simulink model "transientStability_R2013B"  (R2013b)
settings: Solver=ode4  SolverMode=SingleTasking  StartTime=0.0  StopTime=10  FixedStep=0.01  MaxStep=0.01  RelTol=1e-3  AbsTol=1e-2
undefined symbols (not defined in the file): j, mpc
(part 1 of 4)
settings Model: ExtModeTrigMode=oneshot  ExtModeArmWhenConnect=off  Creator=aithal  LastModifiedBy=gelli
settings SolverCC: InitialStep=0.001
settings DataIOCC: LimitDataPoints=off  SignalLoggingSaveFormat=ModelDataLogs  SaveOutput=off  SaveTime=off
settings OptimizationCC: BlockReduction=off  BooleanDataType=off
settings DebuggingCC: SaveWithParameterizedLinksMsg=none  SignalResolutionControl=TryResolveAllWithWarning  SolverPrmCheckMsg=none  MultiTaskDSMMsg=warning  MultiTaskCondExecSysMsg=none  FrameProcessingCompatibilityMsg=error  StateNameClashWarn=warning
settings HardwareCC: TargetUnknown=on
settings GRTTargetCC: CodeReplacementLibrary=C89/C90 (ANSI)  CombineOutputUpdateFcns=off  GRTInterface=on

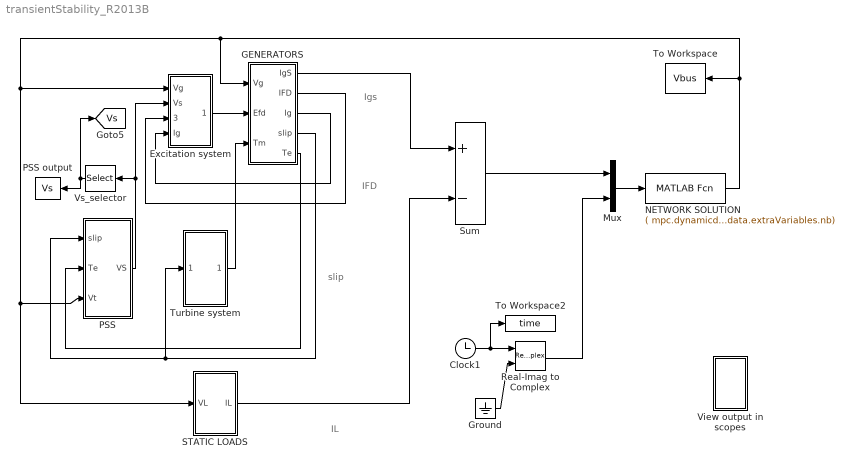
== system transientStability_R2013B ==
  note: Igs
  note: IL
  note: IFD
  note: slip
  Clock1 : Clock
  Excitation system : Subsystem
  GENERATORS : Subsystem
  Ground : Ground
  Mux : Mux  Inputs=[mpc.dynamicdata.extraVariables.nb 1]
  NETWORK SOLUTION : MATLABFcn  MATLABFcn="( mpc.dynamicdata.Yform.Y  * (abs(u(mpc.dynamicdata.extraVariables.nb+1))<mpc.dynamicdata.Yform.Tfault)  + mpc.dynamicdata.Yform.Yf  * (abs(u(mpc.dynamicdata.extraVariables.nb+1))>=mpc.dynamicdata.Yform.Tfault & abs(u(mpc.dynamicdata.extraVariables.nb+1)) <(mpc.dynamicdata.Yform.Tfault+mpc.dynamicdata.Yform.Tclear) ) + mpc.dynamicdata.Yform.Ypf * (abs(u(mpc.dynamicdata.extraVariables.nb+1)) >= (mpc.dynamicdata.Yform.Tfault+mpc.dynamicdata.Yform.Tclear) )  ) \\   u(1:mpc.dynamicdata.extraVariables.nb)"  OutputDimensions=mpc.dynamicdata.extraVariables.nb  OutputSignalType=complex
  PSS : Subsystem
  PSS output : ToWorkspace  VariableName=Vs  SampleTime=0.01
  Real-Imag to Complex : RealImagToComplex
  STATIC LOADS : Subsystem
  Sum : Sum  Inputs=+-  SaturateOnIntegerOverflow=on  InputSameDT=on  OutDataTypeStr=Inherit: Same as first input
  To Workspace : ToWorkspace  VariableName=Vbus  SampleTime=0.01
  To Workspace2 : ToWorkspace  VariableName=time  SampleTime=0.01
  Turbine system : Subsystem
  View output in scopes : Subsystem
  Vs_selector : Selector  InputPortWidth=mpc.dynamicdata.extraVariables.nb  IndexOptions=Index vector (dialog)  Indices=(mpc.dynamicdata.gen(:,1))  OutputSizes=1
  tag scope: Vs=global
  wires:
  Excitation system/1(Efd) -> GENERATORS/2(Efd)
  GENERATORS/2(IFD) -> Excitation system/3(IFD)
  GENERATORS/3(Ig) -> Excitation system/4(Ig)
  GENERATORS/1(IgS) -> Sum/1
  GENERATORS/4(slip) -> Turbine system/1(slip), PSS/1(slip)
  GENERATORS/5(Te) -> PSS/2(Te)
  Sum/1 -> Mux/1
  Ground/1 -> Real-Imag to Complex/2
  Real-Imag to Complex/1 -> Mux/2
  Clock1/1 -> Real-Imag to Complex/1, To Workspace2/1
  Mux/1 -> NETWORK SOLUTION/1
  Turbine system/1(Tm) -> GENERATORS/3(Tm)
  PSS/1(VS) -> Excitation system/2(Vs), Vs_selector/1
  Vs_selector/1 -> PSS output/1, [Vs]
  NETWORK SOLUTION/1 -> GENERATORS/1(Vg), Excitation system/1(Vg), STATIC LOADS/1(VL), PSS/3(Vt), To Workspace/1
  STATIC LOADS/1(IL) -> Sum/2

== system transientStability_R2013B/Excitation system ==
  Vg : Inport
  Vs : Inport  Port=2
  IFD : Inport  Port=3
  Ig : Inport  Port=4
  "Exciter_AC1A " : Subsystem
  Exciter_AC4A : Subsystem
  Exciter_DC1A : Subsystem
  Exciter_ST1A : Subsystem
  Exciter_ST2A : Subsystem
  Exciter_static : Subsystem
  Select-AVR : Subsystem
  Sum1 : Sum  Inputs=++++++  SaturateOnIntegerOverflow=on  InputSameDT=on  OutDataTypeStr=Inherit: Same as first input
  flag : Constant  Value=mpc.dynamicdata.gen_exciterParameters.AVR
  Efd : Outport  InitialOutput=0
  wires:
  Vg/1 -> Exciter_static/1(V), Exciter_DC1A/1(V), Exciter_AC4A/1(V), Exciter_ST2A/1(V), "Exciter_AC1A "/1(V), Exciter_ST1A/1(V)
  Vs/1 -> Exciter_static/2(Vs), Exciter_DC1A/2(Vs), Exciter_AC4A/2(Vs), Exciter_ST2A/2(Vs), "Exciter_AC1A "/2(Vs), Exciter_ST1A/2(Vs)
  Exciter_static/1(Efd) -> Sum1/1
  Exciter_DC1A/1(Efd) -> Sum1/2
  Exciter_AC4A/1(Efd) -> Sum1/3
  Ig/1 -> Exciter_ST2A/4(Ia)
  Exciter_ST2A/1(Efd) -> Sum1/4
  IFD/1 -> Exciter_AC4A/3(IFD), Exciter_ST2A/3(IFD), "Exciter_AC1A "/3(IFD), Exciter_ST1A/3(IFD)
  "Exciter_AC1A "/1(Efd) -> Sum1/5
  Select-AVR/1(out_1) -> Efd/1
  Sum1/1 -> Select-AVR/2(in_2)
  flag/1 -> Select-AVR/1(in_1)
  Exciter_ST1A/1(Efd) -> Sum1/6

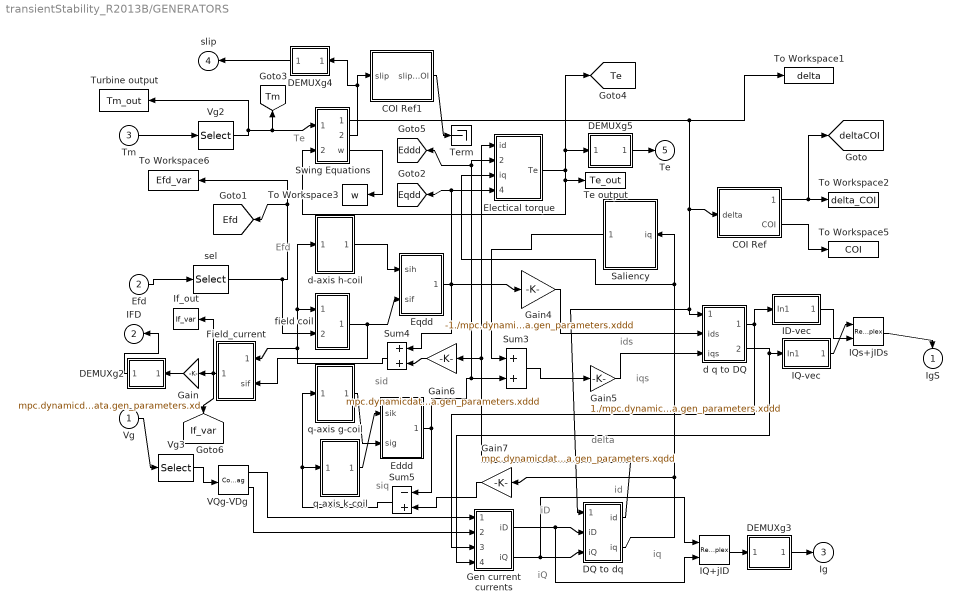
== system transientStability_R2013B/GENERATORS ==
  note: iq
  note: id
  note: Efd
  note: Te
  note: sid
  note: siq
  note: iqs
  note: ids
  note: iD
  note: iQ
  note: delta
  Vg : Inport
  Efd : Inport  Port=2
  Tm : Inport  Port=3
  " field coil" : Subsystem
  COI Ref : Subsystem
  COI Ref1 : Subsystem
  DEMUXg2 : Subsystem
  DEMUXg3 : Subsystem
  DEMUXg4 : Subsystem
  DEMUXg5 : Subsystem
  DQ to dq : Subsystem
  Eddd : Subsystem
  Electical torque : Subsystem
  "Eqdd " : Subsystem
  Field_current : Subsystem
  Gain : Gain  Gain=mpc.dynamicdata.gen_parameters.xd  SaturateOnIntegerOverflow=on  OutDataTypeStr=Inherit: Same as input  ParamDataTypeStr=Inherit: Same as input
  Gain4 : Gain  Gain=-1./mpc.dynamicdata.gen_parameters.xddd  SaturateOnIntegerOverflow=on  OutDataTypeStr=Inherit: Same as input  ParamDataTypeStr=Inherit: Same as input
  Gain5 : Gain  Gain=1./mpc.dynamicdata.gen_parameters.xddd  SaturateOnIntegerOverflow=on  OutDataTypeStr=Inherit: Same as input  ParamDataTypeStr=Inherit: Same as input
  Gain6 : Gain  Gain=mpc.dynamicdata.gen_parameters.xddd  SaturateOnIntegerOverflow=on  OutDataTypeStr=Inherit: Same as input  ParamDataTypeStr=Inherit: Same as input
  Gain7 : Gain  Gain=mpc.dynamicdata.gen_parameters.xqdd  SaturateOnIntegerOverflow=on  OutDataTypeStr=Inherit: Same as input  ParamDataTypeStr=Inherit: Same as input
  Gen current currents : Subsystem
  ID-vec : Subsystem
  IQ+jID : RealImagToComplex
  IQ-vec : Subsystem
  IQs+jIDs : RealImagToComplex
  If_out : ToWorkspace  VariableName=If_var  SampleTime=0.01
  Saliency : Subsystem
  Sum3 : Sum  SaturateOnIntegerOverflow=on  InputSameDT=on  OutDataTypeStr=Inherit: Same as first input
  Sum4 : Sum  SaturateOnIntegerOverflow=on  InputSameDT=on  OutDataTypeStr=Inherit: Same as first input
  Sum5 : Sum  Inputs=-+  SaturateOnIntegerOverflow=on  InputSameDT=on  OutDataTypeStr=Inherit: Same as first input
  Swing Equations : Subsystem
  Te output : ToWorkspace  VariableName=Te_out  SampleTime=0.01
  Term : Terminator
  To Workspace1 : ToWorkspace  VariableName=delta  SampleTime=0.01
  To Workspace2 : ToWorkspace  VariableName=delta_COI  SampleTime=0.01
  To Workspace3 : ToWorkspace  VariableName=w  SampleTime=0.01
  To Workspace5 : ToWorkspace  VariableName=COI  SampleTime=0.01
  To Workspace6 : ToWorkspace  VariableName=Efd_var  SampleTime=0.01
  Turbine output : ToWorkspace  VariableName=Tm_out  SampleTime=0.01
  VQg-VDg : ComplexToRealImag
  Vg2 : Selector  InputPortWidth=mpc.dynamicdata.extraVariables.nb  IndexOptions=Index vector (dialog)  Indices=(mpc.dynamicdata.gen(:,1))  OutputSizes=1
  Vg3 : Selector  InputPortWidth=mpc.dynamicdata.extraVariables.nb  IndexOptions=Index vector (dialog)  Indices=(mpc.dynamicdata.gen(:,1))  OutputSizes=1
  d q to DQ : Subsystem
  d-axis h-coil : Subsystem
  q-axis g-coil : Subsystem
  q-axis k-coil : Subsystem
  sel : Selector  InputPortWidth=mpc.dynamicdata.extraVariables.nb  IndexOptions=Index vector (dialog)  Indices=(mpc.dynamicdata.gen(:,1))  OutputSizes=1
  IgS : Outport  InitialOutput=0
  IFD : Outport  Port=2  InitialOutput=0
  Ig : Outport  Port=3  InitialOutput=0
  slip : Outport  Port=4  InitialOutput=0
  Te : Outport  Port=5  InitialOutput=0
  tag scope: Eddd=global, Efd=global, Eqdd=global, If_var=global, Te=global, Tm=global, deltaCOI=global
  wires:
  Saliency/1(Edumdd) -> Sum3/1
  Sum3/1 -> Gain5/1
  Gain5/1 -> d q to DQ/3(iqs)
  Electical torque/1(Te) -> Swing Equations/2(Te), Te output/1, DEMUXg5/1(In1), [Te]
  Gain4/1 -> d q to DQ/2(ids)
  COI Ref1/1(slip_COI) -> Term/1
  COI Ref/2(COI) -> To Workspace5/1
  COI Ref/1(delta_COI) -> To Workspace2/1, [deltaCOI]
  d-axis h-coil/1(sih) -> "Eqdd "/1(sih)
  q-axis g-coil/1(sig) -> Eddd/2(sig)
  q-axis k-coil/1(sik) -> Eddd/1(sik)
  Gain6/1 -> Sum4/2
  DQ to dq/1(id) -> Electical torque/1(id), Gain6/1
  DQ to dq/2(iq) -> Gain7/1, Saliency/1(iq), Electical torque/3(iq)
  Gain7/1 -> Sum5/2
  Sum5/1 -> q-axis k-coil/1(siq), q-axis g-coil/1(siq)
  Eddd/1(Eddd) -> Sum5/1, Sum3/2, Electical torque/2(Eddd), [Eddd]
  "Eqdd "/1(Eqdd) -> Sum4/1, Gain4/1, Electical torque/4(Eqdd), [Eqdd]
  IQ-vec/1(Out1) -> IQs+jIDs/1
  ID-vec/1(Out1) -> IQs+jIDs/2
  d q to DQ/2(iQs) -> Gen current currents/4(iQs), IQ-vec/1(In1)
  d q to DQ/1(iDs) -> Gen current currents/3(iDs), ID-vec/1(In1)
  IQs+jIDs/1 -> IgS/1
  VQg-VDg/1 -> Gen current currents/1(VQ)
  VQg-VDg/2 -> Gen current currents/2(VD)
  Vg3/1 -> VQg-VDg/1
  Vg/1 -> Vg3/1
  Efd/1 -> sel/1
  Sum4/1 -> " field coil"/1(sid), d-axis h-coil/1(sid), Field_current/1(sid)
  " field coil"/1(sif) -> "Eqdd "/2(sif), Field_current/2(sif)
  Gen current currents/1(iD) -> DQ to dq/2(iD), IQ+jID/2
  Gen current currents/2(iQ) -> DQ to dq/3(iQ), IQ+jID/1
  IQ+jID/1 -> DEMUXg3/1(In1)
  DEMUXg3/1(Out1) -> Ig/1
  Gain/1 -> DEMUXg2/1(In1)
  DEMUXg2/1(Out1) -> IFD/1
  Tm/1 -> Vg2/1
  Swing Equations/2(slip) -> COI Ref1/1(slip), DEMUXg4/1(In1)
  DEMUXg4/1(Out1) -> slip/1
  sel/1 -> To Workspace6/1, [Efd], " field coil"/2(Efd)
  Vg2/1 -> Swing Equations/1(Tm), [Tm], Turbine output/1
  Field_current/1(ifd) -> Gain/1, [If_var], If_out/1
  DEMUXg5/1(Out1) -> Te/1
  Swing Equations/1(delta) -> DQ to dq/1(delta), d q to DQ/1(delta), COI Ref/1(delta), To Workspace1/1
  Swing Equations/3(w) -> To Workspace3/1

== system transientStability_R2013B/PSS ==
  slip : Inport
  Te : Inport  Port=2
  Vt : Inport  Port=3
  Constant : Constant  Value=mpc.dynamicdata.gen_pssParameters.PSS
  PSS_slip_signal : Subsystem
  Power_input_PSS : Subsystem
  Select-PSS : Subsystem
  Sum1 : Sum  Inputs=++++  SaturateOnIntegerOverflow=on  InputSameDT=on  OutDataTypeStr=Inherit: Same as first input
  delP_Omega_PSS : Subsystem
  "frequency_input_PSS " : Subsystem
  VS : Outport
  wires:
  Select-PSS/1(out_1) -> VS/1
  Constant/1 -> Select-PSS/1(in_1)
  PSS_slip_signal/1(vs) -> Sum1/1
  Power_input_PSS/1(Vs) -> Sum1/2
  Sum1/1 -> Select-PSS/2(in_2)
  Vt/1 -> "frequency_input_PSS "/1(V)
  "frequency_input_PSS "/1(Vs) -> Sum1/3
  slip/1 -> PSS_slip_signal/1(slip), delP_Omega_PSS/1(slip)
  Te/1 -> Power_input_PSS/1(Te), delP_Omega_PSS/2(Te)
  delP_Omega_PSS/1(Vs) -> Sum1/4

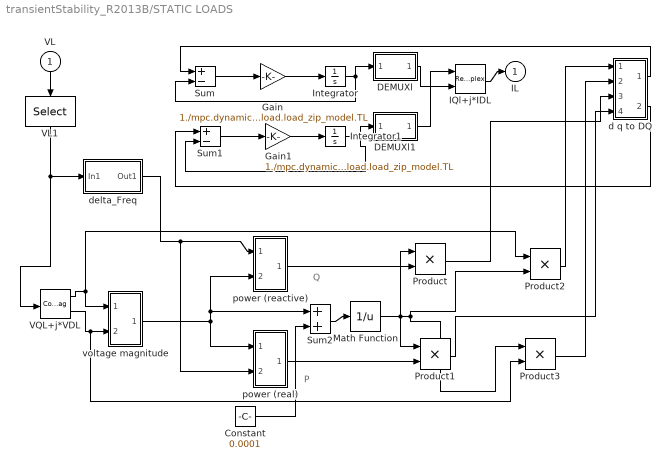
== system transientStability_R2013B/STATIC LOADS ==
  note: P
  note: Q
  VL : Inport
  Constant : Constant  Value=0.0001
  DEMUXl : Subsystem
  DEMUXl1 : Subsystem
  Gain : Gain  Gain=1./mpc.dynamicdata.load.load_zip_model.TL  SaturateOnIntegerOverflow=on  OutDataTypeStr=Inherit: Same as input  ParamDataTypeStr=Inherit: Same as input
  Gain1 : Gain  Gain=1./mpc.dynamicdata.load.load_zip_model.TL  SaturateOnIntegerOverflow=on  OutDataTypeStr=Inherit: Same as input  ParamDataTypeStr=Inherit: Same as input
  IQl+j*IDL : RealImagToComplex
  Integrator : Integrator
  Integrator1 : Integrator
  Math Function : Math  Operator=reciprocal  SaturateOnIntegerOverflow=on
  Product{,1..3} (4 alike) : Product  SaturateOnIntegerOverflow=on  RndMeth=Zero  InputSameDT=on  OutDataTypeStr=Inherit: Same as first input
  Sum : Sum  Inputs=+-  SaturateOnIntegerOverflow=on  InputSameDT=on  OutDataTypeStr=Inherit: Same as first input
  Sum1 : Sum  Inputs=+-  SaturateOnIntegerOverflow=on  InputSameDT=on  OutDataTypeStr=Inherit: Same as first input
  Sum2 : Sum  SaturateOnIntegerOverflow=on  InputSameDT=on  OutDataTypeStr=Inherit: Same as first input
  VL1 : Selector  InputPortWidth=mpc.dynamicdata.extraVariables.nb  IndexOptions=Index vector (dialog)  Indices=(mpc.dynamicdata.extraVariables.ld(:,1))  OutputSizes=1
  VQL+j*VDL : ComplexToRealImag
  d q to DQ : Subsystem
  delta_Freq : Subsystem
  power (reactive) : Subsystem
  power (real) : Subsystem
  voltage magnitude : Subsystem
  IL : Outport  InitialOutput=0
  wires:
  voltage magnitude/1(out_1) -> power (real)/1(in_1), Sum2/1, power (reactive)/2(in_1)
  VQL+j*VDL/1 -> voltage magnitude/1(in_1), Product2/1
  Product2/1 -> d q to DQ/1(in_1)
  Product3/1 -> d q to DQ/2(in_4)
  d q to DQ/1(out_1) -> Sum/1
  d q to DQ/2(out_2) -> Sum1/1
  Product/1 -> d q to DQ/3(in_2)
  Product1/1 -> d q to DQ/4(in_3)
  power (real)/1(out_2) -> Product1/2
  power (reactive)/1(out_1) -> Product/1
  Sum/1 -> Gain/1
  Sum1/1 -> Gain1/1
  Math Function/1 -> Product2/2, Product3/1, Product1/1, Product/2
  Sum2/1 -> Math Function/1
  Constant/1 -> Sum2/2
  VQL+j*VDL/2 -> voltage magnitude/2(in_2), Product3/2
  Integrator/1 -> Sum/2, DEMUXl/1(In1)
  DEMUXl1/1(Out1) -> IQl+j*IDL/1
  DEMUXl/1(Out1) -> IQl+j*IDL/2
  IQl+j*IDL/1 -> IL/1
  Gain/1 -> Integrator/1
  Gain1/1 -> Integrator1/1
  Integrator1/1 -> DEMUXl1/1(In1), Sum1/2
  delta_Freq/1(Out1) -> power (real)/2(del freq), power (reactive)/1(del freq)
  VL/1 -> VL1/1
  VL1/1 -> delta_Freq/1(In1), VQL+j*VDL/1

== system transientStability_R2013B/Turbine system ==
  slip : Inport
  Non Reheat Steam Turbine : Subsystem
  Select-Turbine : Subsystem
  Sped Gov_Hydro Turbine : Subsystem
  Speed Gov. Reheat Steam Turbine : Subsystem
  Sum1 : Sum  Inputs=+++  SaturateOnIntegerOverflow=on  InputSameDT=on  OutDataTypeStr=Inherit: Same as first input
  To Workspace : ToWorkspace  VariableName=Tm  SampleTime=0.01
  flag1 : Constant  Value=mpc.dynamicdata.gen_turbineParameters.TURB
  Tm : Outport  InitialOutput=0
  wires:
  Sped Gov_Hydro Turbine/1(Tm) -> Sum1/1
  Non Reheat Steam Turbine/1(Tm) -> Sum1/2
  slip/1 -> Sped Gov_Hydro Turbine/1(slip), Non Reheat Steam Turbine/1(slip), Speed Gov. Reheat Steam Turbine/1(slip)
  Speed Gov. Reheat Steam Turbine/1(Tm) -> Sum1/3
  flag1/1 -> Select-Turbine/1(in_1)
  Sum1/1 -> Select-Turbine/2(in_2)
  Select-Turbine/1(out_1) -> To Workspace/1, Tm/1

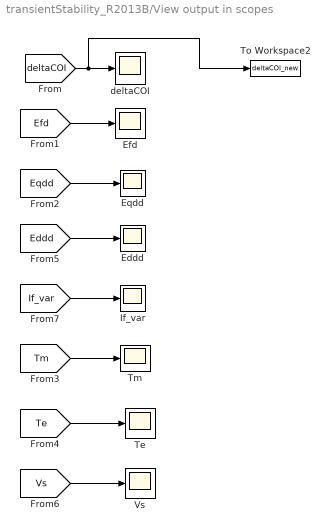
== system transientStability_R2013B/View output in scopes ==
  " Eddd" : Scope
      settings: TimeRange=5  MaxDataPoints=5000  SaveToWorkspace=off  SaveName=ScopeData  YMin=-0.77325  YMax=0.08592  SampleTime=-1
  " Eqdd" : Scope
      settings: TimeRange=5  MaxDataPoints=5000  SaveToWorkspace=off  SaveName=ScopeData  YMin=0.7568  YMax=1.40655  SampleTime=-1
  " If_var" : Scope
      settings: TimeRange=5  MaxDataPoints=5000  SaveToWorkspace=off  SaveName=ScopeData  YMin=-245.34539  YMax=2209.20869  SampleTime=-1
  Efd : Scope
      settings: TimeRange=3  MaxDataPoints=5000  SaveToWorkspace=off  SaveName=ScopeData  YMin=-8.98625  YMax=10.87625  SampleTime=-1
  Te : Scope
      settings: TimeRange=auto  ShowLegends=on  LimitDataPoints=on  MaxDataPoints=5000  SaveToWorkspace=off  SaveName=ScopeData  YMin=-71.17144  YMax=641.63523  SampleTime=-1
  Tm : Scope
      settings: TimeRange=5  MaxDataPoints=5000  SaveToWorkspace=off  SaveName=ScopeData  YMin=-70.795  YMax=639.355  SampleTime=-1
  To Workspace2 : ToWorkspace  VariableName=deltaCOI_new  SampleTime=0.01
  Vs : Scope
      settings: TimeRange=auto  LimitDataPoints=on  MaxDataPoints=5000  SaveToWorkspace=off  SaveName=ScopeData  YMin=-1.00000  YMax=1.00000  SampleTime=-1
  deltaCOI : Scope
      settings: TimeRange=auto  MaxDataPoints=5000  SaveToWorkspace=off  SaveName=ScopeData  YMin=-0.4595  YMax=0.53926  SampleTime=-1
  wires:
  [deltaCOI] -> To Workspace2/1, deltaCOI/1
  [Efd] -> Efd/1
  [Eqdd] -> " Eqdd"/1
  [Eddd] -> " Eddd"/1
  [Tm] -> Tm/1
  [Te] -> Te/1
  [Vs] -> Vs/1
  [If_var] -> " If_var"/1

== system transientStability_R2013B/Excitation system/Exciter_AC1A  ==
  V : Inport
  Vs : Inport  Port=2
  IFD : Inport  Port=3
  Comp to Mag : ComplexToMagnitudeAngle
  DEMUXg2 : Subsystem
  Exciter AC1A : Subsystem
  Select-AVR : Subsystem
  Selector1 : Selector  InputPortWidth=mpc.dynamicdata.extraVariables.nb  IndexOptions=Index vector (dialog)  Indices=mpc.dynamicdata.exc_AC1A(:,1)  OutputSizes=1
  Selector2 : Selector  InputPortWidth=mpc.dynamicdata.extraVariables.nb  IndexOptions=Index vector (dialog)  Indices=mpc.dynamicdata.exc_AC1A(:,1)  OutputSizes=1
  Selector3 : Selector  InputPortWidth=mpc.dynamicdata.extraVariables.nb  IndexOptions=Index vector (dialog)  Indices=mpc.dynamicdata.exc_AC1A(:,1)  OutputSizes=1
  Term : Terminator
  flag : Constant  Value=mpc.dynamicdata.gen_exciterParameters.SL_AC1A
  Efd : Outport
  wires:
  IFD/1 -> Selector3/1
  Selector3/1 -> Exciter AC1A/3(IFD)
  Vs/1 -> Selector2/1
  Selector2/1 -> Exciter AC1A/2(Vs)
  Comp to Mag/2 -> Term/1
  Selector1/1 -> Comp to Mag/1
  V/1 -> Selector1/1
  Comp to Mag/1 -> Exciter AC1A/1(Vg)
  Exciter AC1A/1(Out1) -> DEMUXg2/1(In1)
  flag/1 -> Select-AVR/1(in_1)
  DEMUXg2/1(Out1) -> Select-AVR/2(in_2)
  Select-AVR/1(out_1) -> Efd/1

== system transientStability_R2013B/Excitation system/Exciter_AC4A ==
  V : Inport
  Vs : Inport  Port=2
  IFD : Inport  Port=3
  Comp to Mag : ComplexToMagnitudeAngle
  DEMUXg2 : Subsystem
  Exciter_AC4A : Subsystem
  Select-AVR : Subsystem
  Selector1 : Selector  InputPortWidth=mpc.dynamicdata.extraVariables.nb  IndexOptions=Index vector (dialog)  Indices=mpc.dynamicdata.exc_AC4A(:,1)  OutputSizes=1
  Selector2 : Selector  InputPortWidth=mpc.dynamicdata.extraVariables.nb  IndexOptions=Index vector (dialog)  Indices=mpc.dynamicdata.exc_AC4A(:,1)  OutputSizes=1
  Selector3 : Selector  InputPortWidth=mpc.dynamicdata.extraVariables.nb  IndexOptions=Index vector (dialog)  Indices=mpc.dynamicdata.exc_AC4A(:,1)  OutputSizes=1
  Term : Terminator
  flag : Constant  Value=mpc.dynamicdata.gen_exciterParameters.SL_AC4A
  Efd : Outport
  wires:
  Comp to Mag/2 -> Term/1
  Selector1/1 -> Comp to Mag/1
  V/1 -> Selector1/1
  Comp to Mag/1 -> Exciter_AC4A/1(Vg)
  Exciter_AC4A/1(Out1) -> DEMUXg2/1(In1)
  Vs/1 -> Selector2/1
  Selector2/1 -> Exciter_AC4A/2(Vs)
  IFD/1 -> Selector3/1
  Selector3/1 -> Exciter_AC4A/3(IFD)
  flag/1 -> Select-AVR/1(in_1)
  DEMUXg2/1(Out1) -> Select-AVR/2(in_2)
  Select-AVR/1(out_1) -> Efd/1

== system transientStability_R2013B/Excitation system/Exciter_DC1A ==
  V : Inport
  Vs : Inport  Port=2
  Comp to Mag : ComplexToMagnitudeAngle
  DEMUXg2 : Subsystem
  Select-AVR : Subsystem
  Selector1 : Selector  InputPortWidth=mpc.dynamicdata.extraVariables.nb  IndexOptions=Index vector (dialog)  Indices=mpc.dynamicdata.exc_DC1A(:,1)  OutputSizes=1
  Selector2 : Selector  InputPortWidth=mpc.dynamicdata.extraVariables.nb  IndexOptions=Index vector (dialog)  Indices=mpc.dynamicdata.exc_DC1A(:,1)  OutputSizes=1
  Subsystem : Subsystem
  Term : Terminator
  flag : Constant  Value=mpc.dynamicdata.gen_exciterParameters.SL_DC1A
  Efd : Outport
  wires:
  Comp to Mag/2 -> Term/1
  Selector1/1 -> Comp to Mag/1
  Comp to Mag/1 -> Subsystem/1(Vg)
  Selector2/1 -> Subsystem/2(Vs)
  V/1 -> Selector1/1
  Vs/1 -> Selector2/1
  Subsystem/1(Efd) -> DEMUXg2/1(In1)
  flag/1 -> Select-AVR/1(in_1)
  DEMUXg2/1(Out1) -> Select-AVR/2(in_2)
  Select-AVR/1(out_1) -> Efd/1

== system transientStability_R2013B/Excitation system/Exciter_ST1A ==
  V : Inport
  Vs : Inport  Port=2
  IFD : Inport  Port=3
  Comp to Mag : ComplexToMagnitudeAngle
  DEMUXg2 : Subsystem
  Select-AVR : Subsystem
  Selector1 : Selector  InputPortWidth=mpc.dynamicdata.extraVariables.nb  IndexOptions=Index vector (dialog)  Indices=mpc.dynamicdata.exc_ST1A(:,1)  OutputSizes=1
  Selector2 : Selector  InputPortWidth=mpc.dynamicdata.extraVariables.nb  IndexOptions=Index vector (dialog)  Indices=mpc.dynamicdata.exc_ST1A(:,1)  OutputSizes=1
  Selector3 : Selector  InputPortWidth=mpc.dynamicdata.extraVariables.nb  IndexOptions=Index vector (dialog)  Indices=mpc.dynamicdata.exc_ST1A(:,1)  OutputSizes=1
  Term : Terminator
  delay1 : Subsystem
  exc_ST1A : Subsystem
  flag : Constant  Value=mpc.dynamicdata.gen_exciterParameters.SL_ST1A
  Efd : Outport
  wires:
  Comp to Mag/2 -> Term/1
  Selector1/1 -> Comp to Mag/1
  V/1 -> Selector1/1
  Vs/1 -> Selector2/1
  Selector2/1 -> exc_ST1A/2(Vs)
  IFD/1 -> Selector3/1
  exc_ST1A/1(out_1) -> DEMUXg2/1(In1)
  Selector3/1 -> exc_ST1A/3(IFD)
  Comp to Mag/1 -> delay1/1(Vin)
  delay1/1(Out1) -> exc_ST1A/1(Vg)
  flag/1 -> Select-AVR/1(in_1)
  DEMUXg2/1(Out1) -> Select-AVR/2(in_2)
  Select-AVR/1(out_1) -> Efd/1

== system transientStability_R2013B/Excitation system/Exciter_ST2A ==
  V : Inport
  Vs : Inport  Port=2
  IFD : Inport  Port=3
  Ia : Inport  Port=4
  DEMUXg2 : Subsystem
  ST2A_Exciter : Subsystem
  Select-AVR : Subsystem
  Selector{1..4} (4 alike) : Selector  InputPortWidth=mpc.dynamicdata.extraVariables.nb  IndexOptions=Index vector (dialog)  Indices=mpc.dynamicdata.exc_ST2A(:,1)  OutputSizes=1
  flag : Constant  Value=mpc.dynamicdata.gen_exciterParameters.SL_ST2A
  Efd : Outport
  wires:
  ST2A_Exciter/1(Efd) -> DEMUXg2/1(In1)
  IFD/1 -> Selector4/1
  Vs/1 -> Selector2/1
  Ia/1 -> Selector3/1
  Selector2/1 -> ST2A_Exciter/4(Vs)
  Selector4/1 -> ST2A_Exciter/1(IFD)
  V/1 -> Selector1/1
  Selector1/1 -> ST2A_Exciter/3(Vg)
  Selector3/1 -> ST2A_Exciter/2(Ia)
  flag/1 -> Select-AVR/1(in_1)
  DEMUXg2/1(Out1) -> Select-AVR/2(in_2)
  Select-AVR/1(out_1) -> Efd/1

== system transientStability_R2013B/Excitation system/Exciter_static ==
  V : Inport
  Vs : Inport  Port=2
  Comp to Mag : ComplexToMagnitudeAngle
  DEMUXg2 : Subsystem
  Select-AVR : Subsystem
  Selector1 : Selector  InputPortWidth=mpc.dynamicdata.extraVariables.nb  IndexOptions=Index vector (dialog)  Indices=mpc.dynamicdata.exc_static(:,1)  OutputSizes=1
  Selector2 : Selector  InputPortWidth=mpc.dynamicdata.extraVariables.nb  IndexOptions=Index vector (dialog)  Indices=mpc.dynamicdata.exc_static(:,1)  OutputSizes=1
  Term : Terminator
  exc_static : Subsystem
  flag : Constant  Value=mpc.dynamicdata.gen_exciterParameters.SL_static
  Efd : Outport
  wires:
  Comp to Mag/2 -> Term/1
  Selector1/1 -> Comp to Mag/1
  V/1 -> Selector1/1
  Comp to Mag/1 -> exc_static/1(Vg)
  exc_static/1(out_1) -> DEMUXg2/1(In1)
  Vs/1 -> Selector2/1
  Selector2/1 -> exc_static/2(Vs)
  flag/1 -> Select-AVR/1(in_1)
  DEMUXg2/1(Out1) -> Select-AVR/2(in_2)
  Select-AVR/1(out_1) -> Efd/1

== system transientStability_R2013B/Excitation system/Select-AVR ==
  in_1 : Inport
  in_2 : Inport  Port=2
  Efd : Constant  Value=mpc.dynamicdata.gen_exciterParameters.exciterInitialCondition.EFD0
  Switch : Switch  Threshold=1  SaturateOnIntegerOverflow=on  InputSameDT=on
  out_1 : Outport  InitialOutput=0
  wires:
  in_2/1 -> Switch/3
  in_1/1 -> Switch/2
  Switch/1 -> out_1/1
  Efd/1 -> Switch/1

== system transientStability_R2013B/GENERATORS/ field coil ==
  sid : Inport
  Efd : Inport  Port=2
  Gain : Gain  Gain=1./mpc.dynamicdata.gen_parameters.Tdd  SaturateOnIntegerOverflow=on  OutDataTypeStr=Inherit: Same as input  ParamDataTypeStr=Inherit: Same as input
  Gain1 : Gain  Gain=mpc.dynamicdata.gen_parameters.xdd./(mpc.dynamicdata.gen_parameters.xd-mpc.dynamicdata.gen_parameters.xdd)  SaturateOnIntegerOverflow=on  OutDataTypeStr=Inherit: Same as input  ParamDataTypeStr=Inherit: Same as input
  Integrator2 : Integrator  InitialCondition=mpc.dynamicdata.gen_parameters.sif0
  Sum : Sum  Inputs=+-  SaturateOnIntegerOverflow=on  InputSameDT=on  OutDataTypeStr=Inherit: Same as first input
  Sum1 : Sum  SaturateOnIntegerOverflow=on  InputSameDT=on  OutDataTypeStr=Inherit: Same as first input
  sif : Outport  InitialOutput=0
  wires:
  Efd/1 -> Gain1/1
  Integrator2/1 -> sif/1, Sum/2
  Sum/1 -> Gain/1
  Gain/1 -> Integrator2/1
  sid/1 -> Sum1/1
  Gain1/1 -> Sum1/2
  Sum1/1 -> Sum/1

== system transientStability_R2013B/GENERATORS/COI Ref ==
  delta : Inport
  Gain6 : Gain  Gain=mpc.dynamicdata.gen_parameters.H/sum(mpc.dynamicdata.gen_parameters.H)  SaturateOnIntegerOverflow=on  OutDataTypeStr=Inherit: Same as input  ParamDataTypeStr=Inherit: Same as input
  Sum : Sum  Inputs=+  SaturateOnIntegerOverflow=on  InputSameDT=on  OutDataTypeStr=Inherit: Same as first input
  Sum1 : Sum  Inputs=+-  SaturateOnIntegerOverflow=on  InputSameDT=on  OutDataTypeStr=Inherit: Same as first input
  delta_COI : Outport  InitialOutput=0
  COI : Outport  Port=2  InitialOutput=0
  wires:
  Sum/1 -> Sum1/2, COI/1
  Gain6/1 -> Sum/1
  delta/1 -> Gain6/1, Sum1/1
  Sum1/1 -> delta_COI/1

== system transientStability_R2013B/GENERATORS/COI Ref1 ==
  slip : Inport
  Gain6 : Gain  Gain=mpc.dynamicdata.gen_parameters.H/sum(mpc.dynamicdata.gen_parameters.H)  SaturateOnIntegerOverflow=on  OutDataTypeStr=Inherit: Same as input  ParamDataTypeStr=Inherit: Same as input
  Sum : Sum  Inputs=+  SaturateOnIntegerOverflow=on  InputSameDT=on  OutDataTypeStr=Inherit: Same as first input
  Sum1 : Sum  Inputs=+-  SaturateOnIntegerOverflow=on  InputSameDT=on  OutDataTypeStr=Inherit: Same as first input
  slip_COI : Outport  InitialOutput=0
  wires:
  Sum1/1 -> slip_COI/1
  slip/1 -> Gain6/1, Sum1/1
  Gain6/1 -> Sum/1
  Sum/1 -> Sum1/2

== system transientStability_R2013B/GENERATORS/DEMUXg2 ==
  In1 : Inport
  Dummy Zeros : Constant  Value=zeros(1,mpc.dynamicdata.extraVariables.nb-mpc.dynamicdata.extraVariables.ngen)
  Mux1 : Mux  Inputs=[mpc.dynamicdata.extraVariables.nb-mpc.dynamicdata.extraVariables.ngen mpc.dynamicdata.extraVariables.ngen]
  Selector4 : Selector  InputPortWidth=mpc.dynamicdata.extraVariables.nb  IndexOptions=Index vector (dialog)  Indices=mpc.dynamicdata.gen_parameters.order_gen  OutputSizes=1
  Out1 : Outport
  wires:
  In1/1 -> Mux1/2
  Selector4/1 -> Out1/1
  Dummy Zeros/1 -> Mux1/1
  Mux1/1 -> Selector4/1

== system transientStability_R2013B/GENERATORS/DEMUXg3 ==
  In1 : Inport
  Dummy Zeros : Constant  Value=zeros(1,mpc.dynamicdata.extraVariables.nb-mpc.dynamicdata.extraVariables.ngen)
  IQ+jID : RealImagToComplex
  Mux1 : Mux  Inputs=[mpc.dynamicdata.extraVariables.nb-mpc.dynamicdata.extraVariables.ngen mpc.dynamicdata.extraVariables.ngen]
  Selector4 : Selector  InputPortWidth=mpc.dynamicdata.extraVariables.nb  IndexOptions=Index vector (dialog)  Indices=mpc.dynamicdata.gen_parameters.order_gen  OutputSizes=1
  Out1 : Outport
  wires:
  Mux1/1 -> Selector4/1
  Dummy Zeros/1 -> IQ+jID/2, IQ+jID/1
  Selector4/1 -> Out1/1
  In1/1 -> Mux1/2
  IQ+jID/1 -> Mux1/1

== system transientStability_R2013B/GENERATORS/DEMUXg4 ==
  In1 : Inport
  Dummy Zeros : Constant  Value=zeros(1,mpc.dynamicdata.extraVariables.nb-mpc.dynamicdata.extraVariables.ngen)
  Mux1 : Mux  Inputs=[mpc.dynamicdata.extraVariables.nb-mpc.dynamicdata.extraVariables.ngen mpc.dynamicdata.extraVariables.ngen]
  Selector4 : Selector  InputPortWidth=mpc.dynamicdata.extraVariables.nb  IndexOptions=Index vector (dialog)  Indices=mpc.dynamicdata.gen_parameters.order_gen  OutputSizes=1
  Out1 : Outport
  wires:
  Mux1/1 -> Selector4/1
  Dummy Zeros/1 -> Mux1/1
  Selector4/1 -> Out1/1
  In1/1 -> Mux1/2

== system transientStability_R2013B/GENERATORS/DEMUXg5 ==
  In1 : Inport
  Dummy Zeros : Constant  Value=zeros(1,mpc.dynamicdata.extraVariables.nb-mpc.dynamicdata.extraVariables.ngen)
  Mux1 : Mux  Inputs=[mpc.dynamicdata.extraVariables.nb-mpc.dynamicdata.extraVariables.ngen mpc.dynamicdata.extraVariables.ngen]
  Selector4 : Selector  InputPortWidth=mpc.dynamicdata.extraVariables.nb  IndexOptions=Index vector (dialog)  Indices=mpc.dynamicdata.gen_parameters.order_gen  OutputSizes=1
  Out1 : Outport
  wires:
  In1/1 -> Mux1/2
  Selector4/1 -> Out1/1
  Dummy Zeros/1 -> Mux1/1
  Mux1/1 -> Selector4/1

== system transientStability_R2013B/GENERATORS/DQ to dq ==
  note: I_Q
  note: I_D
  delta : Inport
  iD : Inport  Port=2
  iQ : Inport  Port=3
  Product{,1..3} (4 alike) : Product  SaturateOnIntegerOverflow=on  RndMeth=Zero  InputSameDT=on  OutDataTypeStr=Inherit: Same as first input
  Sum1 : Sum  Inputs=+-  SaturateOnIntegerOverflow=on  InputSameDT=on  OutDataTypeStr=Inherit: Same as first input
  Sum2 : Sum  SaturateOnIntegerOverflow=on  InputSameDT=on  OutDataTypeStr=Inherit: Same as first input
  cos : Trigonometry  Operator=cos
  sin : Trigonometry
  id : Outport  InitialOutput=0
  iq : Outport  Port=2  InitialOutput=0
  wires:
  cos/1 -> Product3/2, Product/2
  sin/1 -> Product2/2, Product1/2
  iD/1 -> Product2/1, Product/1
  iQ/1 -> Product3/1, Product1/1
  Product3/1 -> Sum2/2
  Product2/1 -> Sum2/1
  Product1/1 -> Sum1/2
  Product/1 -> Sum1/1
  delta/1 -> sin/1, cos/1
  Sum1/1 -> id/1
  Sum2/1 -> iq/1

== system transientStability_R2013B/GENERATORS/Eddd ==
  sik : Inport
  sig : Inport  Port=2
  Gain2 : Gain  Gain=1./mpc.dynamicdata.gen_parameters.xqd  SaturateOnIntegerOverflow=on  OutDataTypeStr=Inherit: Same as input  ParamDataTypeStr=Inherit: Same as input
  Gain3 : Gain  Gain=mpc.dynamicdata.gen_parameters.xqdd./(mpc.dynamicdata.gen_parameters.xq.*mpc.dynamicdata.gen_parameters.xqd)  SaturateOnIntegerOverflow=on  OutDataTypeStr=Inherit: Same as input  ParamDataTypeStr=Inherit: Same as input
  Gain4 : Gain  Gain=-1  SaturateOnIntegerOverflow=on  OutDataTypeStr=Inherit: Same as input  ParamDataTypeStr=Inherit: Same as input
  Prod1 : Product  SaturateOnIntegerOverflow=on  RndMeth=Zero  InputSameDT=on  OutDataTypeStr=Inherit: Same as first input
  Prod2 : Product  SaturateOnIntegerOverflow=on  RndMeth=Zero  InputSameDT=on  OutDataTypeStr=Inherit: Same as first input
  Sum3 : Sum  Inputs=+-  SaturateOnIntegerOverflow=on  InputSameDT=on  OutDataTypeStr=Inherit: Same as first input
  Sum4 : Sum  Inputs=+-  SaturateOnIntegerOverflow=on  InputSameDT=on  OutDataTypeStr=Inherit: Same as first input
  Sum5 : Sum  SaturateOnIntegerOverflow=on  InputSameDT=on  OutDataTypeStr=Inherit: Same as first input
  xq : Constant  Value=mpc.dynamicdata.gen_parameters.xq
  xqd : Constant  Value=mpc.dynamicdata.gen_parameters.xqd
  xqdd : Constant  Value=mpc.dynamicdata.gen_parameters.xqdd
  Eddd : Outport
  wires:
  sig/1 -> Prod2/2
  sik/1 -> Prod1/2
  Prod2/1 -> Sum5/2
  Prod1/1 -> Sum5/1
  Gain3/1 -> Prod2/1
  Sum4/1 -> Gain3/1
  xqd/1 -> Sum4/2, Sum3/1
  xq/1 -> Sum4/1
  Gain2/1 -> Prod1/1
  Sum3/1 -> Gain2/1
  xqdd/1 -> Sum3/2
  Sum5/1 -> Gain4/1
  Gain4/1 -> Eddd/1

== system transientStability_R2013B/GENERATORS/Electical torque ==
  id : Inport
  Eddd : Inport  Port=2
  iq : Inport  Port=3
  Eqdd : Inport  Port=4
  Gain : Gain  Gain=(mpc.dynamicdata.gen_parameters.xddd-mpc.dynamicdata.gen_parameters.xqdd)  SaturateOnIntegerOverflow=on  OutDataTypeStr=Inherit: Same as input  ParamDataTypeStr=Inherit: Same as input
  Product : Product  SaturateOnIntegerOverflow=on  RndMeth=Zero  InputSameDT=on  OutDataTypeStr=Inherit: Same as first input
  Product1 : Product  SaturateOnIntegerOverflow=on  RndMeth=Zero  InputSameDT=on  OutDataTypeStr=Inherit: Same as first input
  Product2 : Product  SaturateOnIntegerOverflow=on  RndMeth=Zero  InputSameDT=on  OutDataTypeStr=Inherit: Same as first input
  Sum : Sum  Inputs=3  SaturateOnIntegerOverflow=on  InputSameDT=on  OutDataTypeStr=Inherit: Same as first input
  Te : Outport  InitialOutput=0
  wires:
  Product/1 -> Sum/1
  Product1/1 -> Sum/2
  Gain/1 -> Sum/3
  Product2/1 -> Gain/1
  Sum/1 -> Te/1
  iq/1 -> Product2/2, Product1/1
  id/1 -> Product2/1, Product/1
  Eqdd/1 -> Product1/2
  Eddd/1 -> Product/2

== system transientStability_R2013B/GENERATORS/Eqdd  ==
  sih : Inport
  sif : Inport  Port=2
  Gain2 : Gain  Gain=1./mpc.dynamicdata.gen_parameters.xdd  SaturateOnIntegerOverflow=on  OutDataTypeStr=Inherit: Same as input  ParamDataTypeStr=Inherit: Same as input
  Gain3 : Gain  Gain=mpc.dynamicdata.gen_parameters.xddd./(mpc.dynamicdata.gen_parameters.xd.*mpc.dynamicdata.gen_parameters.xdd)  SaturateOnIntegerOverflow=on  OutDataTypeStr=Inherit: Same as input  ParamDataTypeStr=Inherit: Same as input
  Prod1 : Product  SaturateOnIntegerOverflow=on  RndMeth=Zero  InputSameDT=on  OutDataTypeStr=Inherit: Same as first input
  Prod2 : Product  SaturateOnIntegerOverflow=on  RndMeth=Zero  InputSameDT=on  OutDataTypeStr=Inherit: Same as first input
  Sum3 : Sum  Inputs=+-  SaturateOnIntegerOverflow=on  InputSameDT=on  OutDataTypeStr=Inherit: Same as first input
  Sum4 : Sum  Inputs=+-  SaturateOnIntegerOverflow=on  InputSameDT=on  OutDataTypeStr=Inherit: Same as first input
  Sum5 : Sum  SaturateOnIntegerOverflow=on  InputSameDT=on  OutDataTypeStr=Inherit: Same as first input
  xd : Constant  Value=mpc.dynamicdata.gen_parameters.xd
  xdd : Constant  Value=mpc.dynamicdata.gen_parameters.xdd
  xddd : Constant  Value=mpc.dynamicdata.gen_parameters.xddd
  Eqdd : Outport
  wires:
  xddd/1 -> Sum3/2
  Sum3/1 -> Gain2/1
  Gain2/1 -> Prod1/1
  xd/1 -> Sum4/1
  xdd/1 -> Sum3/1, Sum4/2
  Sum4/1 -> Gain3/1
  Gain3/1 -> Prod2/1
  Prod1/1 -> Sum5/1
  Prod2/1 -> Sum5/2
  sih/1 -> Prod1/2
  Sum5/1 -> Eqdd/1
  sif/1 -> Prod2/2

== system transientStability_R2013B/GENERATORS/Field_current ==
  sid : Inport
  sif : Inport  Port=2
  1/xfl : Gain  Gain=1./mpc.dynamicdata.gen_parameters.xfl  SaturateOnIntegerOverflow=on  OutDataTypeStr=Inherit: Same as input  ParamDataTypeStr=Inherit: Same as input
  Sum3 : Sum  Inputs=-+  SaturateOnIntegerOverflow=on  InputSameDT=on  OutDataTypeStr=Inherit: Same as first input
  ifd : Outport
  wires:
  Sum3/1 -> 1/xfl/1
  1/xfl/1 -> ifd/1
  sid/1 -> Sum3/1
  sif/1 -> Sum3/2

== system transientStability_R2013B/GENERATORS/Gen current currents ==
  VQ : Inport
  VD : Inport  Port=2
  iDs : Inport  Port=3
  iQs : Inport  Port=4
  Gain : Gain  Gain=1./mpc.dynamicdata.gen_parameters.xddd  SaturateOnIntegerOverflow=on  OutDataTypeStr=Inherit: Same as input  ParamDataTypeStr=Inherit: Same as input
  Gain1 : Gain  Gain=1./mpc.dynamicdata.gen_parameters.xddd  SaturateOnIntegerOverflow=on  OutDataTypeStr=Inherit: Same as input  ParamDataTypeStr=Inherit: Same as input
  Sum : Sum  SaturateOnIntegerOverflow=on  InputSameDT=on  OutDataTypeStr=Inherit: Same as first input
  Sum2 : Sum  Inputs=+-  SaturateOnIntegerOverflow=on  InputSameDT=on  OutDataTypeStr=Inherit: Same as first input
  iD : Outport  InitialOutput=0
  iQ : Outport  Port=2  InitialOutput=0
  wires:
  Sum/1 -> iD/1
  Sum2/1 -> iQ/1
  Gain1/1 -> Sum2/2
  Gain/1 -> Sum/2
  iDs/1 -> Sum/1
  iQs/1 -> Sum2/1
  VD/1 -> Gain1/1
  VQ/1 -> Gain/1

== system transientStability_R2013B/GENERATORS/ID-vec ==
  In1 : Inport
  Dummy Zeros : Constant  Value=zeros(1,mpc.dynamicdata.extraVariables.nb-mpc.dynamicdata.extraVariables.ngen)
  Mux1 : Mux  Inputs=[mpc.dynamicdata.extraVariables.nb-mpc.dynamicdata.extraVariables.ngen; mpc.dynamicdata.extraVariables.ngen]
  Selector4 : Selector  InputPortWidth=mpc.dynamicdata.extraVariables.nb  IndexOptions=Index vector (dialog)  Indices=mpc.dynamicdata.gen_parameters.order_gen  OutputSizes=1
  Out1 : Outport
  wires:
  Mux1/1 -> Selector4/1
  In1/1 -> Mux1/2
  Dummy Zeros/1 -> Mux1/1
  Selector4/1 -> Out1/1

== system transientStability_R2013B/GENERATORS/IQ-vec ==
  In1 : Inport
  Dummy Zeros : Constant  Value=zeros(1,mpc.dynamicdata.extraVariables.nb-mpc.dynamicdata.extraVariables.ngen)
  Mux1 : Mux  Inputs=[mpc.dynamicdata.extraVariables.nb-mpc.dynamicdata.extraVariables.ngen; mpc.dynamicdata.extraVariables.ngen]
  Selector4 : Selector  InputPortWidth=mpc.dynamicdata.extraVariables.nb  IndexOptions=Index vector (dialog)  Indices=mpc.dynamicdata.gen_parameters.order_gen  OutputSizes=1
  Out1 : Outport
  wires:
  Selector4/1 -> Out1/1
  Dummy Zeros/1 -> Mux1/1
  In1/1 -> Mux1/2
  Mux1/1 -> Selector4/1

== system transientStability_R2013B/GENERATORS/Saliency ==
  iq : Inport
  Gain1 : Gain  Gain=1./mpc.dynamicdata.gen_parameters.Tdummy  SaturateOnIntegerOverflow=on  OutDataTypeStr=Inherit: Same as input  ParamDataTypeStr=Inherit: Same as input
  Gain6 : Gain  Gain=(mpc.dynamicdata.gen_parameters.xddd-mpc.dynamicdata.gen_parameters.xqdd)  SaturateOnIntegerOverflow=on  OutDataTypeStr=Inherit: Same as input  ParamDataTypeStr=Inherit: Same as input
  Integrator1 : Integrator  InitialCondition=mpc.dynamicdata.gen_parameters.Edummydd0
  Sum1 : Sum  Inputs=+-  SaturateOnIntegerOverflow=on  InputSameDT=on  OutDataTypeStr=Inherit: Same as first input
  Edumdd : Outport  InitialOutput=0
  wires:
  Integrator1/1 -> Sum1/2, Edumdd/1
  Sum1/1 -> Gain1/1
  Gain1/1 -> Integrator1/1
  Gain6/1 -> Sum1/1
  iq/1 -> Gain6/1

== system transientStability_R2013B/GENERATORS/Swing Equations ==
  Tm : Inport
  Te : Inport  Port=2
  Gain : Gain  Gain=mpc.dynamicdata.extraVariables.wB  SaturateOnIntegerOverflow=on  OutDataTypeStr=Inherit: Same as input  ParamDataTypeStr=Inherit: Same as input
  Gain1 : Gain  Gain=mpc.dynamicdata.gen_parameters.D  SaturateOnIntegerOverflow=on  OutDataTypeStr=Inherit: Same as input  ParamDataTypeStr=Inherit: Same as input
  Gain2 : Gain  Gain=1/2./mpc.dynamicdata.gen_parameters.H  SaturateOnIntegerOverflow=on  OutDataTypeStr=Inherit: Same as input  ParamDataTypeStr=Inherit: Same as input
  Integrator : Integrator
  Integrator1 : Integrator  InitialCondition=mpc.dynamicdata.gen_parameters.delta0
  Sum1 : Sum  Inputs=+--  SaturateOnIntegerOverflow=on  InputSameDT=on  OutDataTypeStr=Inherit: Same as first input
  delta : Outport  InitialOutput=0
  slip : Outport  Port=2  InitialOutput=0
  w : Outport  Port=3  InitialOutput=0
  wires:
  Gain1/1 -> Sum1/3
  Gain/1 -> w/1, Integrator1/1
  Te/1 -> Sum1/2
  Tm/1 -> Sum1/1
  Gain2/1 -> Integrator/1
  Integrator/1 -> Gain1/1, Gain/1, slip/1
  Integrator1/1 -> delta/1
  Sum1/1 -> Gain2/1

== system transientStability_R2013B/GENERATORS/d q to DQ ==
  note: I_qS
  note: I_dS
  delta : Inport
  ids : Inport  Port=2
  iqs : Inport  Port=3
  Product{,1..3} (4 alike) : Product  SaturateOnIntegerOverflow=on  RndMeth=Zero  InputSameDT=on  OutDataTypeStr=Inherit: Same as first input
  Sum1 : Sum  SaturateOnIntegerOverflow=on  InputSameDT=on  OutDataTypeStr=Inherit: Same as first input
  Sum2 : Sum  Inputs=-+  SaturateOnIntegerOverflow=on  InputSameDT=on  OutDataTypeStr=Inherit: Same as first input
  cos : Trigonometry  Operator=cos
  sin : Trigonometry
  iDs : Outport  InitialOutput=0
  iQs : Outport  Port=2  InitialOutput=0
  wires:
  Sum2/1 -> iQs/1
  Sum1/1 -> iDs/1
  delta/1 -> sin/1, cos/1
  Product/1 -> Sum1/1
  Product1/1 -> Sum1/2
  Product2/1 -> Sum2/1
  Product3/1 -> Sum2/2
  iqs/1 -> Product3/1, Product1/1
  ids/1 -> Product2/1, Product/1
  sin/1 -> Product1/2, Product2/2
  cos/1 -> Product3/2, Product/2

== system transientStability_R2013B/GENERATORS/d-axis h-coil ==
  sid : Inport
  Gain : Gain  Gain=1./mpc.dynamicdata.gen_parameters.Tddd  SaturateOnIntegerOverflow=on  OutDataTypeStr=Inherit: Same as input  ParamDataTypeStr=Inherit: Same as input
  Integrator2 : Integrator  InitialCondition=mpc.dynamicdata.gen_parameters.sih0
  Sum : Sum  Inputs=+-  SaturateOnIntegerOverflow=on  InputSameDT=on  OutDataTypeStr=Inherit: Same as first input
  sih : Outport  InitialOutput=0
  wires:
  Gain/1 -> Integrator2/1
  Sum/1 -> Gain/1
  Integrator2/1 -> Sum/2, sih/1
  sid/1 -> Sum/1

== system transientStability_R2013B/GENERATORS/q-axis g-coil ==
  siq : Inport
  Gain : Gain  Gain=1./mpc.dynamicdata.gen_parameters.Tqd  SaturateOnIntegerOverflow=on  OutDataTypeStr=Inherit: Same as input  ParamDataTypeStr=Inherit: Same as input
  Integrator2 : Integrator  InitialCondition=mpc.dynamicdata.gen_parameters.sig0
  Sum : Sum  Inputs=+-  SaturateOnIntegerOverflow=on  InputSameDT=on  OutDataTypeStr=Inherit: Same as first input
  sig : Outport  InitialOutput=0
  wires:
  siq/1 -> Sum/1
  Integrator2/1 -> sig/1, Sum/2
  Sum/1 -> Gain/1
  Gain/1 -> Integrator2/1

== system transientStability_R2013B/GENERATORS/q-axis k-coil ==
  siq : Inport
  Gain : Gain  Gain=1./mpc.dynamicdata.gen_parameters.Tqdd  SaturateOnIntegerOverflow=on  OutDataTypeStr=Inherit: Same as input  ParamDataTypeStr=Inherit: Same as input
  Integrator2 : Integrator  InitialCondition=mpc.dynamicdata.gen_parameters.sik0
  Sum : Sum  Inputs=+-  SaturateOnIntegerOverflow=on  InputSameDT=on  OutDataTypeStr=Inherit: Same as first input
  sik : Outport  InitialOutput=0
  wires:
  Gain/1 -> Integrator2/1
  Sum/1 -> Gain/1
  Integrator2/1 -> Sum/2, sik/1
  siq/1 -> Sum/1

== system transientStability_R2013B/PSS/PSS_slip_signal ==
  slip : Inport
  Compensator : Subsystem
  Constant : Constant  Value=mpc.dynamicdata.gen_pssParameters.SL_slip_pss
  DEMUXg2 : Subsystem
  FILT(s) : Subsystem
  Gain2 : Gain  Gain=mpc.dynamicdata.gen_pssParameters.pss_slip_signalParameters.Kslip_pss  SaturateOnIntegerOverflow=on  OutDataTypeStr=Inherit: Same as input  ParamDataTypeStr=Inherit: Same as input
  Limiter : Saturate  UpperLimit=mpc.dynamicdata.gen_pssParameters.pss_slip_signalParameters.VS_slip_max  LowerLimit=mpc.dynamicdata.gen_pssParameters.pss_slip_signalParameters.VS_slip_min
  Select-PSS : Subsystem
  Selector1 : Selector  InputPortWidth=mpc.dynamicdata.extraVariables.nb  IndexOptions=Index vector (dialog)  Indices=mpc.dynamicdata.slip_pss(:,1)  OutputSizes=1
  Wash_out : Subsystem
  delay : Subsystem
  vs : Outport
  wires:
  slip/1 -> Selector1/1
  Selector1/1 -> Gain2/1
  Wash_out/1(out) -> Compensator/1(in)
  Limiter/1 -> DEMUXg2/1(In1)
  Compensator/1(Vs) -> FILT(s)/1(In1)
  FILT(s)/1(Vs) -> Limiter/1
  Gain2/1 -> delay/1(Vin)
  delay/1(Out1) -> Wash_out/1(in)
  Constant/1 -> Select-PSS/1(in_1)
  DEMUXg2/1(Out1) -> Select-PSS/2(in_2)
  Select-PSS/1(out_1) -> vs/1

== system transientStability_R2013B/PSS/Power_input_PSS ==
  Te : Inport
  Constant : Constant  Value=mpc.dynamicdata.gen_pssParameters.SL_power_pss
  DEMUXg2 : Subsystem
  Gain2 : Gain  Gain=-mpc.dynamicdata.gen_pssParameters.pss_power_signalParameters.Kpower_pss  SaturateOnIntegerOverflow=on  OutDataTypeStr=Inherit: Same as input  ParamDataTypeStr=Inherit: Same as input
  Limiter : Saturate  UpperLimit=mpc.dynamicdata.gen_pssParameters.pss_power_signalParameters.VS_power_max  LowerLimit=mpc.dynamicdata.gen_pssParameters.pss_power_signalParameters.VS_power_min
  Select-PSS : Subsystem
  Selector1 : Selector  InputPortWidth=mpc.dynamicdata.extraVariables.nb  IndexOptions=Index vector (dialog)  Indices=mpc.dynamicdata.power_pss(:,1)  OutputSizes=1
  Wash_out : Subsystem
  delay1 : Subsystem
  Vs : Outport
  wires:
  Gain2/1 -> Limiter/1
  Te/1 -> Selector1/1
  Limiter/1 -> DEMUXg2/1(In1)
  Selector1/1 -> Wash_out/1(in)
  Wash_out/1(out) -> delay1/1(Vin)
  delay1/1(Out1) -> Gain2/1
  Constant/1 -> Select-PSS/1(in_1)
  DEMUXg2/1(Out1) -> Select-PSS/2(in_2)
  Select-PSS/1(out_1) -> Vs/1

== system transientStability_R2013B/PSS/Select-PSS ==
  in_1 : Inport
  in_2 : Inport  Port=2
  Switch : Switch  Threshold=1  SaturateOnIntegerOverflow=on  InputSameDT=on
  Vs=0 : Constant  Value=zeros(1,mpc.dynamicdata.extraVariables.nb)
  out_1 : Outport  InitialOutput=0
  wires:
  in_2/1 -> Switch/3
  in_1/1 -> Switch/2
  Switch/1 -> out_1/1
  Vs=0/1 -> Switch/1

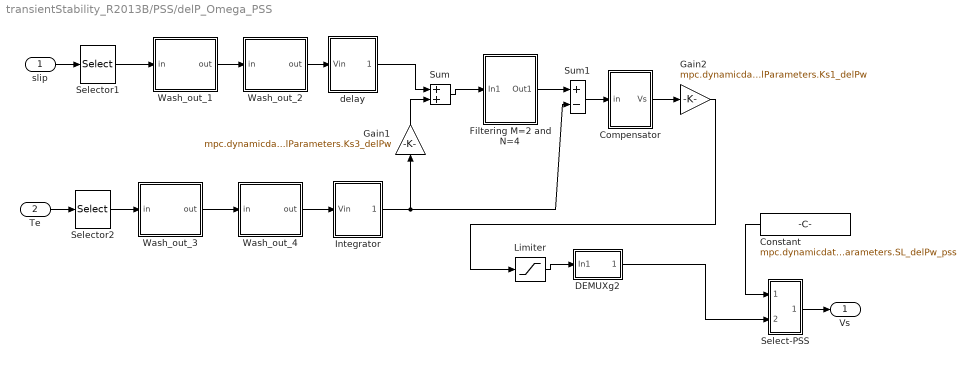
== system transientStability_R2013B/PSS/delP_Omega_PSS ==
  slip : Inport
  Te : Inport  Port=2
  Compensator : Subsystem
  Constant : Constant  Value=mpc.dynamicdata.gen_pssParameters.SL_delPw_pss
  DEMUXg2 : Subsystem
  Filtering M=2 and N=4 : Subsystem
  Gain1 : Gain  Gain=mpc.dynamicdata.gen_pssParameters.pss_delPw_signalParameters.Ks3_delPw  SaturateOnIntegerOverflow=on  OutDataTypeStr=Inherit: Same as input  ParamDataTypeStr=Inherit: Same as input
  Gain2 : Gain  Gain=mpc.dynamicdata.gen_pssParameters.pss_delPw_signalParameters.Ks1_delPw  SaturateOnIntegerOverflow=on  OutDataTypeStr=Inherit: Same as input  ParamDataTypeStr=Inherit: Same as input
  Integrator : Subsystem
  Limiter : Saturate  UpperLimit=mpc.dynamicdata.gen_pssParameters.pss_delPw_signalParameters.VS_delPw_max  LowerLimit=mpc.dynamicdata.gen_pssParameters.pss_delPw_signalParameters.VS_delPw_min
  Select-PSS : Subsystem
  Selector1 : Selector  InputPortWidth=mpc.dynamicdata.extraVariables.nb  IndexOptions=Index vector (dialog)  Indices=mpc.dynamicdata.delPw_pss(:,1)  OutputSizes=1
  Selector2 : Selector  InputPortWidth=mpc.dynamicdata.extraVariables.nb  IndexOptions=Index vector (dialog)  Indices=mpc.dynamicdata.delPw_pss(:,1)  OutputSizes=1
  Sum : Sum  SaturateOnIntegerOverflow=on  InputSameDT=on  OutDataTypeStr=Inherit: Same as first input
  Sum1 : Sum  Inputs=+-  SaturateOnIntegerOverflow=on  InputSameDT=on  OutDataTypeStr=Inherit: Same as first input
  Wash_out_1 : Subsystem
  Wash_out_2 : Subsystem
  Wash_out_3 : Subsystem
  Wash_out_4 : Subsystem
  delay : Subsystem
  Vs : Outport
  wires:
  Wash_out_2/1(out) -> delay/1(Vin)
  Wash_out_1/1(out) -> Wash_out_2/1(in)
  Wash_out_3/1(out) -> Wash_out_4/1(in)
  Wash_out_4/1(out) -> Integrator/1(Vin)
  delay/1(Out1) -> Sum/1
  Gain1/1 -> Sum/2
  Sum/1 -> Filtering M=2 and N=4/1(In1)
  Filtering M=2 and N=4/1(Out1) -> Sum1/1
  Integrator/1(Out1) -> Gain1/1, Sum1/2
  Sum1/1 -> Compensator/1(in)
  Compensator/1(Vs) -> Gain2/1
  Selector1/1 -> Wash_out_1/1(in)
  Selector2/1 -> Wash_out_3/1(in)
  slip/1 -> Selector1/1
  Te/1 -> Selector2/1
  Limiter/1 -> DEMUXg2/1(In1)
  Gain2/1 -> Limiter/1
  Constant/1 -> Select-PSS/1(in_1)
  DEMUXg2/1(Out1) -> Select-PSS/2(in_2)
  Select-PSS/1(out_1) -> Vs/1

== system transientStability_R2013B/PSS/frequency_input_PSS  ==
  V : Inport
  Compensator : Subsystem
  Constant : Constant  Value=mpc.dynamicdata.gen_pssParameters.SL_freq_pss
  DEMUXg2 : Subsystem
  FILT(s) : Subsystem
  Gain2 : Gain  Gain=mpc.dynamicdata.gen_pssParameters.pss_freq_signalParameters.Kfreq_pss  SaturateOnIntegerOverflow=on  OutDataTypeStr=Inherit: Same as input  ParamDataTypeStr=Inherit: Same as input
  Limiter : Saturate  UpperLimit=mpc.dynamicdata.gen_pssParameters.pss_freq_signalParameters.VS_freq_max  LowerLimit=mpc.dynamicdata.gen_pssParameters.pss_freq_signalParameters.VS_freq_min
  Select-PSS : Subsystem
  Selector1 : Selector  InputPortWidth=mpc.dynamicdata.extraVariables.nb  IndexOptions=Index vector (dialog)  Indices=mpc.dynamicdata.freq_pss(:,1)  OutputSizes=1
  Wash_out : Subsystem
  delay : Subsystem
  delta_Freq : Subsystem
  Vs : Outport
  wires:
  V/1 -> Selector1/1
  Selector1/1 -> delta_Freq/1(In1)
  delta_Freq/1(Out1) -> delay/1(Vin)
  delay/1(Out1) -> Wash_out/1(in)
  Gain2/1 -> Limiter/1
  Limiter/1 -> DEMUXg2/1(In1)
  FILT(s)/1(Vs) -> Gain2/1
  Constant/1 -> Select-PSS/1(in_1)
  DEMUXg2/1(Out1) -> Select-PSS/2(in_2)
  Select-PSS/1(out_1) -> Vs/1
  Wash_out/1(out) -> Compensator/1(in)
  Compensator/1(Vs) -> FILT(s)/1(In1)

== system transientStability_R2013B/STATIC LOADS/DEMUXl ==
  In1 : Inport
  Dummy Zeros : Constant  Value=zeros(1,mpc.dynamicdata.extraVariables.nb-mpc.dynamicdata.extraVariables.nload)
  Mux1 : Mux  Inputs=[mpc.dynamicdata.extraVariables.nb-mpc.dynamicdata.extraVariables.nload mpc.dynamicdata.extraVariables.nload]
  Selector4 : Selector  InputPortWidth=mpc.dynamicdata.extraVariables.nb  IndexOptions=Index vector (dialog)  Indices=mpc.dynamicdata.load.load_zip_model.order_load  OutputSizes=1
  Out1 : Outport
  wires:
  In1/1 -> Mux1/2
  Selector4/1 -> Out1/1
  Dummy Zeros/1 -> Mux1/1
  Mux1/1 -> Selector4/1

== system transientStability_R2013B/STATIC LOADS/DEMUXl1 ==
  In1 : Inport
  Dummy Zeros : Constant  Value=zeros(1,mpc.dynamicdata.extraVariables.nb-mpc.dynamicdata.extraVariables.nload)
  Mux1 : Mux  Inputs=[mpc.dynamicdata.extraVariables.nb-mpc.dynamicdata.extraVariables.nload mpc.dynamicdata.extraVariables.nload]
  Selector4 : Selector  InputPortWidth=mpc.dynamicdata.extraVariables.nb  IndexOptions=Index vector (dialog)  Indices=mpc.dynamicdata.load.load_zip_model.order_load  OutputSizes=1
  Out1 : Outport
  wires:
  Mux1/1 -> Selector4/1
  Dummy Zeros/1 -> Mux1/1
  Selector4/1 -> Out1/1
  In1/1 -> Mux1/2

== system transientStability_R2013B/STATIC LOADS/d q to DQ ==
  note: I_P
  note: I_R
  note: cos(delta)
  note: sin(delta)
  in_1 : Inport
  in_4 : Inport  Port=2
  in_2 : Inport  Port=3
  in_3 : Inport  Port=4
  Product{,1..3} (4 alike) : Product  SaturateOnIntegerOverflow=on  RndMeth=Zero  InputSameDT=on  OutDataTypeStr=Inherit: Same as first input
  Sum1 : Sum  Inputs=-+  SaturateOnIntegerOverflow=on  InputSameDT=on  OutDataTypeStr=Inherit: Same as first input
  Sum2 : Sum  SaturateOnIntegerOverflow=on  InputSameDT=on  OutDataTypeStr=Inherit: Same as first input
  out_1 : Outport  InitialOutput=0
  out_2 : Outport  Port=2  InitialOutput=0
  wires:
  Sum2/1 -> out_2/1
  Sum1/1 -> out_1/1
  Product/1 -> Sum1/1
  Product1/1 -> Sum1/2
  Product2/1 -> Sum2/1
  Product3/1 -> Sum2/2
  in_3/1 -> Product3/1, Product1/1
  in_2/1 -> Product2/1, Product/1
  in_4/1 -> Product1/2, Product2/2
  in_1/1 -> Product3/2, Product/2

== system transientStability_R2013B/STATIC LOADS/delta_Freq ==
  In1 : Inport
  Bus_freq : Scope
      settings: TimeRange=3  MaxDataPoints=5000  SaveToWorkspace=off  SaveName=ScopeData  YMin=-0.4  YMax=0.5  SampleTime=-1
  Complex to Magnitude-Angle : ComplexToMagnitudeAngle
  Complex to Real-Imag : ComplexToRealImag
  Math Function : Math  Operator=square  SaturateOnIntegerOverflow=on
  Pref : Constant  Value=0.00001
  Product : Product  SaturateOnIntegerOverflow=on  RndMeth=Zero  InputSameDT=on  OutDataTypeStr=Inherit: Same as first input
  Product1 : Product  SaturateOnIntegerOverflow=on  RndMeth=Zero  InputSameDT=on  OutDataTypeStr=Inherit: Same as first input
  Product2 : Product  Inputs=*/  SaturateOnIntegerOverflow=on  RndMeth=Zero  InputSameDT=on  OutDataTypeStr=Inherit: Same as first input
  Sum : Sum  Inputs=+-  SaturateOnIntegerOverflow=on  InputSameDT=on  OutDataTypeStr=Inherit: Same as first input
  Sum2 : Sum  SaturateOnIntegerOverflow=on  InputSameDT=on  OutDataTypeStr=Inherit: Same as first input
  T 1 : Terminator
  derivative1 : Subsystem
  derivative2 : Subsystem
  Out1 : Outport
  wires:
  Complex to Real-Imag/1 -> Product/2, derivative2/1(In3)
  derivative1/1(Out2) -> Product/1
  Pref/1 -> Sum2/2
  Sum2/1 -> Math Function/1
  Complex to Magnitude-Angle/1 -> Sum2/1
  Product/1 -> Sum/1
  Product1/1 -> Sum/2
  Sum/1 -> Product2/1
  Math Function/1 -> Product2/2
  Complex to Real-Imag/2 -> Product1/1, derivative1/1(In3)
  derivative2/1(Out2) -> Product1/2
  Complex to Magnitude-Angle/2 -> T 1/1
  In1/1 -> Complex to Real-Imag/1, Complex to Magnitude-Angle/1
  Product2/1 -> Out1/1, Bus_freq/1
